simulink model "flightControlSystem"  (Simulink 8.4)
settings: Solver=ode45  StartTime=0.0  StopTime=10.0  RelTol=1e-3
settings Model: Creator=brtaylor  LastModifiedBy=brtaylor
settings DataIOCC: SignalLoggingSaveFormat=Dataset
settings OptimizationCC: ExpressionDepthLimit=128
settings DebuggingCC: UnderspecifiedInitializationDetection=Simplified  MergeDetectMultiDrivingBlocksExec=error  FcnCallInpInsideContextMsg=EnableAllAsError  StateNameClashWarn=none
settings GRTTargetCC: CombineOutputUpdateFcns=on  GRTInterface=off

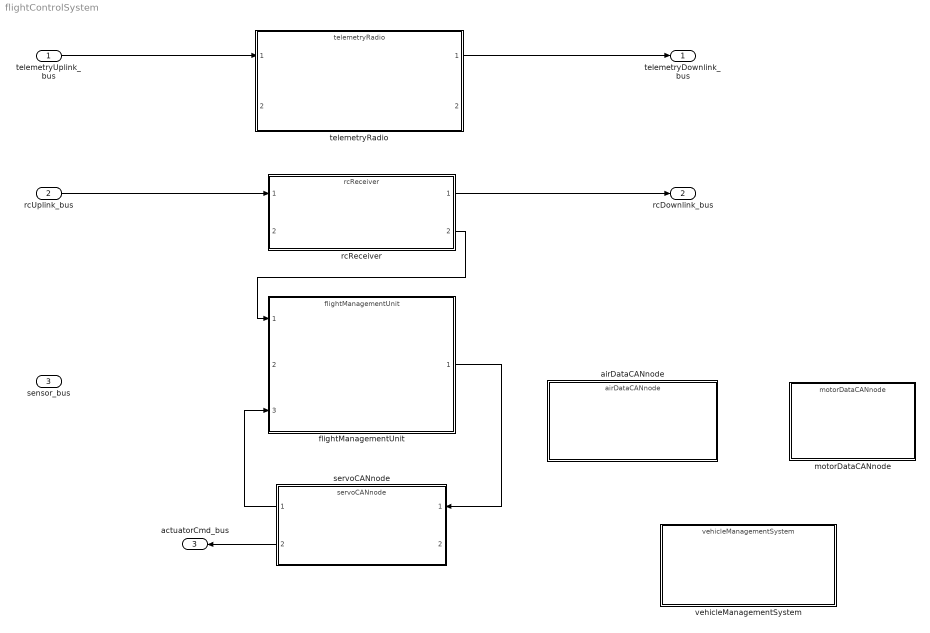
== system flightControlSystem ==
  telemetryUplink_bus : Inport
  rcUplink_bus : Inport  Port=2
  sensor_bus : Inport  Port=3
  airDataCANnode : ModelReference  ModelNameDialog=airDataCANnode.mdl  SimulationMode=Normal  ModelReferenceVersion=1.0  CopyOfModelName=airDataCANnode.mdl  DefaultDataLogging=on
  flightManagementUnit : ModelReference  ModelNameDialog=flightManagementUnit.mdl  SimulationMode=Normal  ModelReferenceVersion=1.3  CopyOfModelName=flightManagementUnit.mdl  DefaultDataLogging=on
  motorDataCANnode : ModelReference  ModelNameDialog=motorDataCANnode.mdl  SimulationMode=Normal  ModelReferenceVersion=1.0  CopyOfModelName=motorDataCANnode.mdl  DefaultDataLogging=on
  rcReceiver : ModelReference  ModelNameDialog=rcReceiver.mdl  SimulationMode=Normal  ModelReferenceVersion=1.2  CopyOfModelName=rcReceiver.mdl  DefaultDataLogging=on
  servoCANnode : ModelReference  ModelNameDialog=servoCANnode.mdl  SimulationMode=Normal  ModelReferenceVersion=1.1  CopyOfModelName=servoCANnode.mdl  DefaultDataLogging=on
  telemetryRadio : ModelReference  ModelNameDialog=telemetryRadio.mdl  SimulationMode=Normal  ModelReferenceVersion=1.1  CopyOfModelName=telemetryRadio.mdl  DefaultDataLogging=on
  vehicleManagementSystem : ModelReference  ModelNameDialog=vehicleManagementSystem.mdl  SimulationMode=Normal  ModelReferenceVersion=1.0  CopyOfModelName=vehicleManagementSystem.mdl  DefaultDataLogging=on
  telemetryDownlink_bus : Outport
  rcDownlink_bus : Outport  Port=2
  actuatorCmd_bus : Outport  Port=3
  wires:
  telemetryUplink_bus/1 -> telemetryRadio/1
  telemetryRadio/1 -> telemetryDownlink_bus/1
  rcUplink_bus/1 -> rcReceiver/1
  rcReceiver/1 -> rcDownlink_bus/1
  rcReceiver/2 -> flightManagementUnit/1
  flightManagementUnit/1 -> servoCANnode/1
  servoCANnode/1 -> flightManagementUnit/3
  servoCANnode/2 -> actuatorCmd_bus/1
